simulink model "rm_project"  (R2024b)
settings: Solver=ode45  StartTime=0.0  StopTime=60  RelTol=1e-3  AbsTol=1e-6
undefined symbols (not defined in the file): sfunxy2
libraries: neural x1, models_lib x1
settings Model: TunableVars=prueba  TunableVarsStorageClass=Auto  Creator=The MathWorks, Inc.  LastModifiedBy=ikostelidis
settings SolverCC: AutoScaleAbsTol=off  AlgebraicLoopSolver=TrustRegion
settings DataIOCC: SaveFormat=Array  SaveOutput=off  ReturnWorkspaceOutputs=off  SignalLoggingName=sigsOut
settings OptimizationCC: BooleanDataType=off  DefaultParameterBehavior=Inlined  ReuseModelBlockBuffer=off  ExpressionDepthLimit=2147483647  InitFltsAndDblsToZero=on  LifeSpan=inf
settings DebuggingCC: SaveWithParameterizedLinksMsg=none  UnderspecifiedInitializationDetection=Classic  MergeDetectMultiDrivingBlocksExec=none  SignalResolutionControl=TryResolveAllWithWarning  MultiTaskDSMMsg=warning  MultiTaskCondExecSysMsg=none  FcnCallInpInsideContextMsg=warning  UnconnectedInputMsg=warning  UnconnectedOutputMsg=warning  UnconnectedLineMsg=warning  StateNameClashWarn=warning  SFUnexpectedBacktrackingDiag=warning  SFNoUnconditionalDefaultTransitionDiag=warning  SFExecutionAtInitializationDiag=none  ArithmeticOperatorsInVariantConditions=warning
settings HardwareCC: ProdBitPerPointer=32  ProdBitPerSizeT=32  ProdBitPerPtrDiffT=32  ProdLargestAtomicFloat=None  ProdIntDivRoundTo=Undefined  ProdEndianess=Unspecified  ProdWordSize=32  ProdHWDeviceType=32-bit Generic  TargetUnknown=on
settings ModelReferenceCC: PropagateSignalLabelsOutOfModel=off
settings SFSimCC: SimUseLocalCustomCode=off  CustomCodeUndefinedFunction=UseInterfaceOnly
settings RTWCC: TemplateMakefile=grt_vc.tmf  RTWUseLocalCustomCode=off  GPUComputeCapability=3.5
settings CodeAppCC: StateflowObjectComments=on
settings GRTTargetCC: TargetFcnLib=ansi_tfl_tmw.mat  TargetLangStandard=C89/C90 (ANSI)  CombineOutputUpdateFcns=off  GRTInterface=on
settings ConfigComp: CovMetricSettings=dw  CovSaveCumulativeToWorkspaceVar=on  CovSaveSingleToWorkspaceVar=on  CovExternalEMLEnable=off

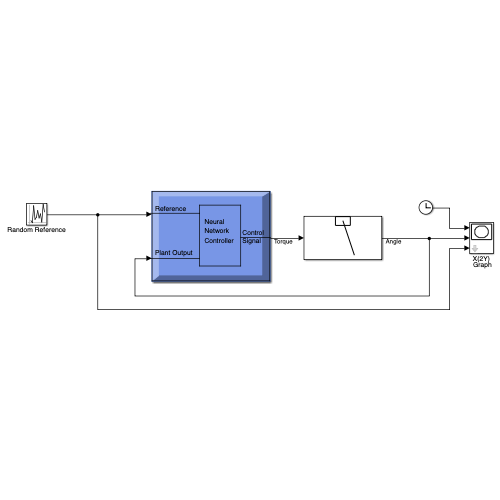
[thumbnail: Simulink's stored preview of the top-level diagram]
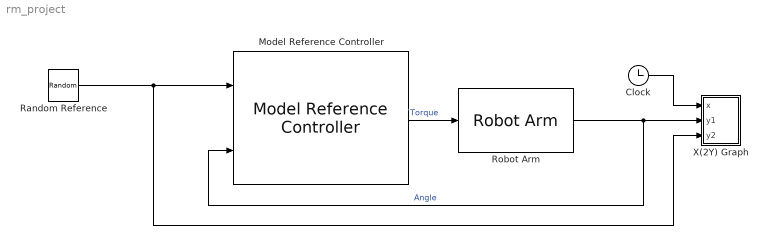
== system rm_project ==
  Clock : Clock
  Model Reference Controller : neural/Control Systems/Model Reference Controller  Nrc=15  Nic=10  Njc=35  IW_y=[0.045509970098621940759 0.31268642922106359983 0.15720134780955610787 0.20798945824301931506 0.29782790203620634895 0.054823120978052183871 0.071206178459122138058 -0.18227893311391640818 0.051855560405362745302 0.3602459537135066503 -0.26021557946947987405 -0.026725443931453655294 -0.14768076980051542124 -0.11447940555067905033 0.17630875982389554446 0.41293266752003143782 0.045482677377962410503 0.16261830351767805891 0.012409568545813482246 0.096914298390607014899 0.15333866355517875024 -0.14469222948698551301 0.25150681247449296896 0.033176627688299667462 0.16737010565516868832 0.14974141731536305677 0.11110059935009626575 0.44729994921254789819 0.014585804033841841612 0.48628418962238428858 0.31475818464290744592 0.53128313219130962608 0.21663990088607507078 -0.07976947470521553174 0.40460905233840149808;0.31490577121449975229 -0.070090923037151267594 -0.13739615264867141575 -0.26489396313576069053 0.20595193039061926443 0.26535665681937342653 -0.020532687345697030884 0.21264607799896900753 0.028610885615719238578 0.1733922806315315035 -0.20442199902699678682 0.018324098953126324862 0.20389427440621374354 -0.21791041570469885102 -0.1464859638823361454 -0.0063664756367045475041 -0.23967882443728244501 -0.090836714019678119203 -0.13314566706521002715 0.19972901273233428787 -0.17880531142350347684 0.077026863598138886613 0.21666720316133822322 -0.12229472194581732236 0.13854147465370894587 -0.20687341064484224273 0.081334477019122664032 -0.10816626919671272489 -0.35025346429988862829 -0.090323739102681988022 -0.32839261606012370986 -0.16007773972217753666 0.032373214828442652136 -0.18131464099604052698 -0.25749991019590268149;-0.074583346114825324613 -0.15272402150577710223 0.21178380027384047235 -0.052927766710515959658 0.24371204015658354258 0.013012514198145018821 0.17912613082950640253 0.21468213259100857315 0.18397193136077452658 -0.1402255253481000663 0.26960202840909214261 0.028206794033129499455 -0.37271856735452824072 0.10397403943177899177 0.13076325797369339754 -0.30425797375280316803 -0.097169105807382805118 -0.17726403343937241486 0.41741114873817036779 0.1823357883450709982 0.33943669839426088286 -0.1415401935814995793 0.0019029470919455912167 -0.051928345312906826203 0.063549167173117093732 -0.058232239761121698529 -0.068420196795155485692 -0.18832040341517439219 0.21375213179171068112 -0.10700029562629104207 -0.28737205353847583567 -0.048670679056887398983 -0.074258173162307095083 0.28737448664363518525 0.13303581980414524999;0.032171040951568412314 0.13600528199919229011 0.23022785348505592218 0.16353264879837170476 0.081051972130842059316 0.42645390483049350205 -0.086597821453507153877 0.30439248493696929865 0.39733246694500273799 -0.18758468453199228509 0.18105349792153951904 -0.011580227993568767419 -0.0050875896031338345427 -0.21566269334153062576 -0.14529181164934243387 0.29642940714458992923 -0.059585942860313365066 0.26148331692843218566 -0.14459665443308922228 -0.16598337395299114783 -0.049483307644019217109 -0.20783733105599225266 -0.057851024777519570452 0.26291939158510635455 -0.13043227427695161524 0.23880479071358423626 -0.094698012545692988873 -0.1707671804510519642 -0.061047513296924448001 0.22028355259459683757 0.26015123889184771366 -0.10837494972468507404 0.04977664980755899804 0.15216443791675166031 0.0050893698285245040497;-0.013291370976571407342 -0.30836282690379535065 0.10878724721595214864 -0.21840087816807818299 0.16846966333389096215 0.092350596645047799971 -0.0099308801531400765772 0.097588491237693544833 0.32758992213034893171 0.25160813442215262947 -0.28247738823506229888 0.18243554890880378516 0.38355253481657425318 0.32988499503674273416 0.22817839363941017083 -0.029156015663233621205 0.16474853956609986083 -0.14172828582141883125 -0.28889093691514888818 -0.49828078647113593913 0.025106439426068570542 -0.11753578179227705536 -0.30152964727798353683 -0.17347424000739886107 0.1604276777534437981 -0.38416345550892772032 0.023898444300467048401 0.16907552827282362751 ...(+2661 chars)]  IW_u=[-0.34526922800968157246 0.37067182761800321344 -0.22842586876992107547 0.34271225995250736984 -0.25157738940466234379 0.37473167224213316251 0.05689179171739792984 0.25179967934526470419 0.23010722369203376325 0.61465893627251178;0.65506217460529359009 0.21523458102448778106 0.30519135272425196304 0.14670807050479869882 0.036949992652394146597 0.47750221075896065459 -0.078303342243597001682 0.14248814163352727102 0.21079974671742099379 0.19344393183071253994;-0.21390828840168846225 -0.11165471261267227721 -0.20254492543232471835 0.0022789695532827031199 0.14293778818775748629 0.13881652460959345574 0.19272863230975931237 0.012079874105486713975 0.039529682040044658575 0.097217728755142326924;-0.18426048661178925925 -0.20033450048398607213 0.13922646158776585956 -0.05316103010121785849 -0.099951028421143811586 0.0042832810066741689239 -0.13317401319369046031 0.085775421783833447065 0.18831370014791978806 0.083908261112988588581;-0.1268448965143226248 -0.34729740023820721007 -0.3341332039885287486 0.076104769947962030985 0.32335786090631668532 0.095742786276205360529 0.27569520477251913126 0.026792936191127436629 -0.095901564991002594129 -0.053214400504005034132;0.047035539991040167807 -0.078517093593909084714 -0.051668000621016868523 0.29177731766714026795 0.35666185145209211571 0.10549301332219469807 0.097614784593004058633 -0.15092956862936993123 -0.036554950544553523051 -0.0049457728287304811299;0.1342543500537145551 0.16908710654609382384 0.16507967020741329267 0.16388575489195228441 0.1329129005312771894 0.03587326848858023165 0.064142181994346722518 0.017356144571413930494 -0.0067652649999094868066 0.014366360542436795028;0.1298238422857348473 -0.55428589636838265786 -0.38511429445782130454 -0.22943877257369377221 0.36325620463834384921 0.40590194985217892265 0.23934299133549960525 0.018710376074039192229 -0.067161052688216427153 0.1332890772646594113]  IW_r=[-0.098808526694725784534 -0.026161860914494561997 -0.23812236124222768696 0.045071572640471214977 -0.3662911448121696778 -0.11300384694224908932 -0.06993499100747738173 -0.020433645010240572559 -0.30937743185481147989 0.041634856502062701777 0.13490069657176800844 0.070523465522609754541 0.17326160845279123257 -0.15757311972672741196 -0.025242468326138911561;0.65509937732438783264 0.56254906260847192812 0.27018403900395432382 0.43199264431004824605 -0.076084900532905383463 -0.028284167083726937525 0.21279428091866467443 0.42548782297787673956 -0.054833475180335475296 0.19228367987128203165 -0.12256255834689511186 0.18392150769260282028 0.19765066127904626359 -0.20812435770282952663 0.28123280201014444479;1.8576070104928417148 0.082618861071812044194 -0.2024699380391932757 -0.62234630799555679115 -0.05739901499883734437 -0.30410331939013296454 -0.41448097676297246394 0.19981511540976104602 -0.20125355005972711542 -0.3339711905692154259 -0.20193765875532207477 -0.33863714114465942595 -0.14873744787613193963 -0.49388437525451450716 -0.43765478905763544049;1.5663574463678611171 -0.014107123599073246797 -0.15154271386049647519 -0.12104562412566285956 -0.11238317796595602427 -0.48506676715100000008 -0.3435263646014739547 -0.3322415832899857091 -0.15547822810255856885 -0.085379084378367192665 -0.26794669218128663868 -0.4206606754486652 -0.31764884729718495526 0.090669340513142140936 -0.052447765479552495294;1.9061142967156528005 0.64394907424290925846 0.025071015461092679977 -0.21818740972705827352 -0.059384349409325874747 0.029798887620237263923 -0.25947117674827085976 -0.32898642563146662798 0.31051685000015222249 0.12154139028521604438 -0.028651433965923883002 -0.36088148532726638251 -0.20511941565987801273 0.15017424838892814987 -0.1804808611957319231;-1.3989544200468109203 -0.48456368261932974972 0.12751735576582223786 0.36617560681922872723 0.31830842243393481228 -0.18131148691322676592 -0.17812922225535993137 -0.016078747566967224042 -0.71115266058357251566 -0.66628532882347468735 -0.59879245949567649898 0.0014021734781582751751 -0.06732123384756480422 0.091078295495689839956 0.11030253757972412199;-2.5474352691341928256 -1.0304149195280611906 -0.18768591806673512457 -0.35400427411211365936 -0.50736377689640443922 -0.45162282359693506351 -0.49637251909572011055 -0.61654250879607130909 -0.52675482721971311761 -0.52211474765588727909 -0.56666383663669261939 -0.33065421468665301408 -0.28991536556736396957 0.07558972585015853729 -0.24934583689141717744;-0.711316890791583889 -0.0087481370761118039392 -0.26841775062293771192 0.29331628630662970325 -0.2372617387820012691 0.10778087559549438812 -0.24673395001757600364 -0.00262699207025781983 -0.012604845555718297706 -0.013020991502317559932 0.062985051719844947771 -0.0082733862496441983037 -0.15718692641729387072 0.13987571335341356105 0.01183867055606833453]  B1_c=[-1.3263182834218101291;-0.93943730369873923447;-0.047698421880223565439;0.10007349383528751918;-0.041170685939811393905;-0.33610193376821073663;0.013579398870262451848;1.1122447799285786196]  B2_c=-0.14872458925088941073  LW_c=[-0.041169806009262420454 -0.071690874054168796103 2.9191991273267690055 2.0953552828240575856 2.5634220160559020307 -2.5838257512082072331 -4.8281315370205604154 -0.82090999492476213195]  retraining_c=10  max_i_int=2  min_i_int=0.1  max_r_int=3  min_r_int=2  Ts=0.1  S1=10  Ni=2  Nj=4  sim_file=robotarm  trainfun=trainlm  Use_validation=1  Use_Testing=1  Use_Inc_training=0  Use_previous_weights=1  max_i=4  min_i=-4  max_r=4  min_r=-4  sam_training=10000  sam_training_c=2000  epochs=300  epochs_c=10  minp=-3.9952396601416353406  maxp=3.9956630319336721158  mint=-1.2553619219262504014  maxt=3.9956630319336721158  Normalize=0  IW=[0.0030145621111318764151 0.0064456179019094644866;0.14706484383143589301 0.093469978878742601691;0.0027593253501936496584 0.0029621343028977879623;-0.0031067513211305371364 -0.0017206268015148051039;-0.27361833701779131323 -0.20525555593630345763;-0.020987299108962693961 -0.040253630664754729007;-0.0042710561030570252244 -0.0060409326207327956187;-0.0051090186413207784935 0.0077011785236896189433;-0.0057919917573147324322 -0.0062994826934297965676;0.0006834965402757509122 0.0076908467839712172515]  LW1_2=[0.51366012870612853813 -0.034194616745323792861 0.27183018874299796908 -0.18549179704118734513;0.20125195326174113997 0.3794258917187361968 0.8731372782914309516 0.15401170249756240826;0.47167494239206314566 0.2617685213117094678 -0.48092803446433385339 0.1821207804768888161;-0.43069441414097969778 0.75051564555945693424 -0.44292923790698085496 0.14831892960058648545;-0.30821817791691530353 0.11215450172368052195 0.57956937274600739407 -0.88884566814974652615;-0.44528391765826180748 -0.88183567775841953384 -0.15550882344036823235 0.57965803982706565201;-0.4762318069017716371 -0.34635094551871187241 0.50344984636474265915 -0.15692812304238351606;-0.76598226100116595383 -0.012353687963619101528 0.50873755453482794042 -0.28523671054343613385;-0.97031636495960327249 1.1219986560873131953 -0.50920924556395585903 0.16763781156855298016;0.25519884518863322764 0.61380698063755945171 -0.44615061803023614573 0.094433239084380921069]  LW2_1=[0.67620928528821488968 -1.1872774877203464395e-05 1.5170109307143795352 -1.7975709460799020878 1.3838223076926505158e-06 -0.0068603685790701611144 -0.65610378107027256256 -0.44915197204848755774 -0.55111574688558351287 1.1604952326387341088]  B1=[-1.7298875717853470224;-1.2030027320349596653;-0.8893858983199430801;0.25798219337965955233;0.3270722456362289976;0.60280431498068620666;-0.24940297304511876986;-1.2610590131842738248;-1.2886314195990755671;1.4349650030174585513]  B2=0.11918451390822200342  S1c=8  Limit_output=0  min_output=-3.1  max_output=3.1  Ref_file=robotref
  Random Reference : UniformRandomNumber  Minimum=-0.8  Maximum=0.8  SampleTime=2
  Robot Arm : models_lib/Robot Arm  SystemSampleTime=-1  VariantActivationTime=update diagram  AllowFlexibleInterface=on  Latency=0  AutoFrameSizeCalculation=off
  X(2Y) Graph : Subsystem  LoadFcn=sfunxy2([],[],[],'LoadBlock')  StartFcn=sfunxy2([],[],[],'Start')  StopFcn=sfunxy2([],[],[],'Stop')  mask(X(2Y) scope.){xmin=0, xmax=60, ymin=-1, ymax=1, st=-1}
      mask prompts: xmin "x-min:"; xmax "x-max:"; ymin "y-min:"; ymax "y-max:"; st "Sample time:"
      mask help: X(2Y) scope using MATLAB graph window. First input is used as time base. Enter plotting ranges.
      settings: CopyFcn=sfunxy2([],[],[],'CopyBlock')  DeleteFcn=sfunxy2([],[],[],'DeleteBlock')  NameChangeFcn=sfunxy2([],[],[],'NameChange')
      mask Help: This block can be used to explore limit cycles. Look at the function sfunxy.m to see how it works.
      mask Display: plot([.05 .95 .95 .05 .05],[.45 .45 .95 .95 .45], 0.5+cos(0:0.1:2*pi)*0.3,0.7+sin(0:0.1:2*pi)*0.2)
  wires:
  Robot Arm/1 -> X(2Y) Graph/2(y1), Model Reference Controller/2  "Angle"
  Model Reference Controller/1 -> Robot Arm/1  "Torque"
  Clock/1 -> X(2Y) Graph/1(x)
  Random Reference/1 -> X(2Y) Graph/3(y2), Model Reference Controller/1

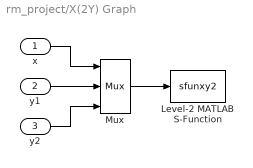
== system rm_project/X(2Y) Graph ==
  x : Inport
  y1 : Inport  Port=2
  y2 : Inport  Port=3
  Level-2 MATLAB S-Function : M-S-Function  FunctionName=sfunxy2  Parameters=[xmin xmax ymin ymax], st
  Mux : Mux  Inputs=3
  wires:
  y2/1 -> Mux/3
  y1/1 -> Mux/2
  x/1 -> Mux/1
  Mux/1 -> Level-2 MATLAB S-Function/1
